simulink model "ControlSemCanalslx"  (Simulink 7.2)
settings: Solver=ode1  StartTime=0.0  StopTime=2  FixedStep=Ts  RelTol=1e-3
values from neighbouring files (symbols this model uses):
  C = [1 0]    [PIexp1.mat]    (also in PIexp3.mat; PIexp4.mat; PIpertubado.mat; ProjetoControlPI.m = GYzss.C)
  F = [621.187048977 29.8812144134]    [PIexp1.mat]    (also in PIexp3.mat; PIexp4.mat; PIpertubado.mat; ProjetoControlPI.m = FKi(1:size(G,2)))
  G = [1  0.0120914439825; 0  0.863556887172]    [PIexp1.mat]    (also in PIexp3.mat; PIexp4.mat; PIpertubado.mat; ProjetoControlPI.m = GYzss.A)
  H = [9.60922939797e-05 0.014430735648]    [PIexp1.mat]    (also in PIexp3.mat; PIexp4.mat; PIpertubado.mat; ProjetoControlPI.m = GYzss.B)
  K_AMP = 1    [PIexp1.mat]    (also in PIexp3.mat; PIexp4.mat; PIpertubado.mat; SemCanalExp1.mat)
  K_EC = 2.27485440932e-05    [PIexp1.mat]    (also in PIexp3.mat; PIexp4.mat; PIpertubado.mat; SemCanalExp1.mat)
  K_EP = 0.00153398078789    [PIexp1.mat]    (also in PIexp3.mat; PIexp4.mat; PIpertubado.mat; SemCanalExp1.mat)
  Kc = 1    [PIexp1.mat]    (also in PIexp3.mat; PIexp4.mat; PIpertubado.mat; ProjetoControlPI.m = 1/Y(end))
  L = [1.86355688717 61.6742300141]    [PIexp1.mat]    (also in PIexp3.mat; PIexp4.mat; PIpertubado.mat; ProjetoControlPI.m = L')
  Ts = 0.013    [PIexp1.mat]    (also in PIexp3.mat; PIexp4.mat; PIpertubado.mat; ProjetoControlPI.m)
  VMAX_AMP = 12    [PIexp1.mat]    (also in PIexp3.mat; PIexp4.mat; PIpertubado.mat; SemCanalExp1.mat)
  VMAX_DAC = 10    [PIexp1.mat]    (also in PIexp3.mat; PIexp4.mat; PIpertubado.mat; SemCanalExp1.mat)
  X_LIM_ENABLE = 1    [PIexp1.mat]    (also in PIexp3.mat; PIexp4.mat; PIpertubado.mat; SemCanalExp1.mat)
  X_MAX = 0.3    [PIexp1.mat]    (also in PIexp3.mat; PIexp4.mat; PIpertubado.mat; SemCanalExp1.mat)
  X_MIN = -0.3    [PIexp1.mat]    (also in PIexp3.mat; PIexp4.mat; PIpertubado.mat; SemCanalExp1.mat)
undefined symbols (not defined in the file or in its folder): HIL, qc_get_step_size
libraries: quarc_library x5, simulink x2, simulink_extras x1
settings Model: Creator=castr  LastModifiedBy=Aluno  SimulationMode=external  CovMetricSettings=dwe  CovHtmlReporting=off  covSaveCumulativeToWorkspaceVar=off  CovSaveSingleToWorkspaceVar=off  ExtModeTrigDuration=50000
settings SolverCC: PositivePriorityOrder=on
settings DataIOCC: LimitDataPoints=off  SaveFormat=StructureWithTime
settings OptimizationCC: ExpressionDepthLimit=128
settings DebuggingCC: UnderspecifiedInitializationDetection=Simplified  MergeDetectMultiDrivingBlocksExec=error  SolverPrmCheckMsg=none  FcnCallInpInsideContextMsg=Enable All  StateNameClashWarn=none  StrictBusMsg=ErrorLevel1
settings HardwareCC: ProdIntDivRoundTo=Zero  ProdEndianess=LittleEndian  ProdHWDeviceType=Specified
settings RTWCC: SystemTargetFile=quarc_windows.tlc  TemplateMakefile=quarc_default_tmf  Description=QUARC Win32 Target  ProcessScript=quarc_windows_make_rtw_hook
settings STFCustomTargetCC: TargetPreCompLibLocation=C:\DOCUME~1\ALLUSE~1\DADOSD~1\QUARC\lib\2008b\windows\release  SystemTargetFile=quarc_windows.tlc
settings GRTTargetCC: TargetPreCompLibLocation=C:\DOCUME~1\ALLUSE~1\DADOSD~1\QUARC\lib\2008b\windows\release  CompOptLevelCompliant=off  MatFileLogging=off  ExtMode=on  ExtModeMexFile=quarc_comm

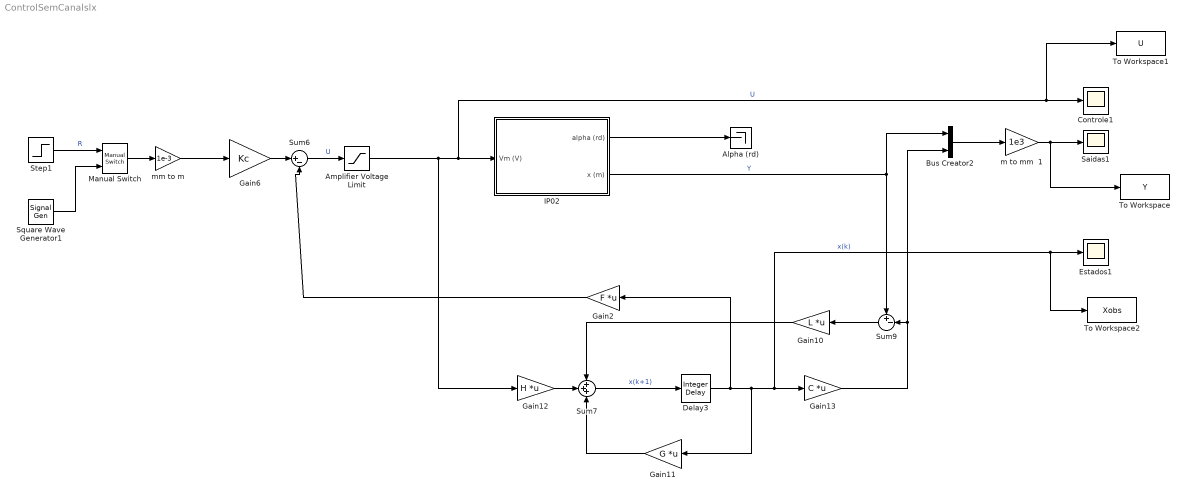
== system ControlSemCanalslx ==
  Alpha (rd) : Terminator
  Amplifier Voltage Limit : Saturate  UpperLimit=VMAX_AMP  LowerLimit=- VMAX_AMP  SampleTime=Ts
  Bus Creator2 : BusCreator  Inputs=2
  Controle1 : Scope
      settings: YMin=-1.5  YMax=13.5
  Delay3 : simulink/Discrete/Integer Delay  vinit=0.0  samptime=Ts  NumDelays=1
  Estados1 : Scope
      settings: YMin=-0.06898  YMax=0.62082  SaveName=ScopeData2
  Gain10 : Gain  Orientation=left  Gain=L  Multiplication=Matrix(K*u)
  Gain11 : Gain  Orientation=left  Gain=G  Multiplication=Matrix(K*u)
  Gain12 : Gain  Gain=H  Multiplication=Matrix(K*u)
  Gain13 : Gain  Gain=C  Multiplication=Matrix(K*u)
  Gain2 : Gain  Orientation=left  Gain=F  Multiplication=Matrix(K*u)
  Gain6 : Gain  Gain=Kc
  IP02 : Subsystem
  Manual Switch : simulink/Signal Routing/Manual Switch  SystemSampleTime=-1  sw=1  action=0  varsize=off
  Saidas1 : Scope
      settings: YMin=-37.5  YMax=337.5  SaveName=ScopeData3
  Square Wave Generator1 : SignalGenerator  WaveForm=square  Amplitude=150  Frequency=1.5  Units=rad/sec
  Step1 : Step  After=15  SampleTime=0
  Sum6 : Sum  Inputs=|+-
  Sum7 : Sum  Inputs=+++
  Sum9 : Sum  Orientation=left  Inputs=+-|
  To Workspace : ToWorkspace  VariableName=Y  SampleTime=-1  SaveFormat=Structure
  To Workspace1 : ToWorkspace  VariableName=U  SampleTime=-1  SaveFormat=Structure
  To Workspace2 : ToWorkspace  VariableName=Xobs  SampleTime=-1  SaveFormat=Structure
  m to mm  1 : Gain  Gain=1e3  SaturateOnIntegerOverflow=on  OutDataTypeStr=Inherit: Same as input  ParamDataTypeStr=Inherit: Same as input
  mm to m : Gain  Gain=1e-3
  wires:
  Gain11/1 -> Sum7/3
  Sum7/1 -> Delay3/1  "x(k+1)"
  Gain10/1 -> Sum7/1
  IP02/2(x (m)) -> Bus Creator2/1, Sum9/1  "Y"
  Amplifier Voltage Limit/1 -> IP02/1(Vm (V)), Controle1/1, To Workspace1/1, Gain12/1  "U"
  Delay3/1 -> Gain2/1, Gain13/1, Estados1/1, To Workspace2/1, Gain11/1  "x(k)"
  Gain12/1 -> Sum7/2
  Gain13/1 -> Sum9/2, Bus Creator2/2
  Sum9/1 -> Gain10/1
  Gain2/1 -> Sum6/2
  mm to m/1 -> Gain6/1
  Manual Switch/1 -> mm to m/1
  Square Wave Generator1/1 -> Manual Switch/2
  Step1/1 -> Manual Switch/1  "R"
  Gain6/1 -> Sum6/1
  Sum6/1 -> Amplifier Voltage Limit/1  "U"
  Bus Creator2/1 -> m to mm  1/1
  m to mm  1/1 -> Saidas1/1, To Workspace/1
  IP02/1(alpha (rd)) -> Alpha (rd)/1

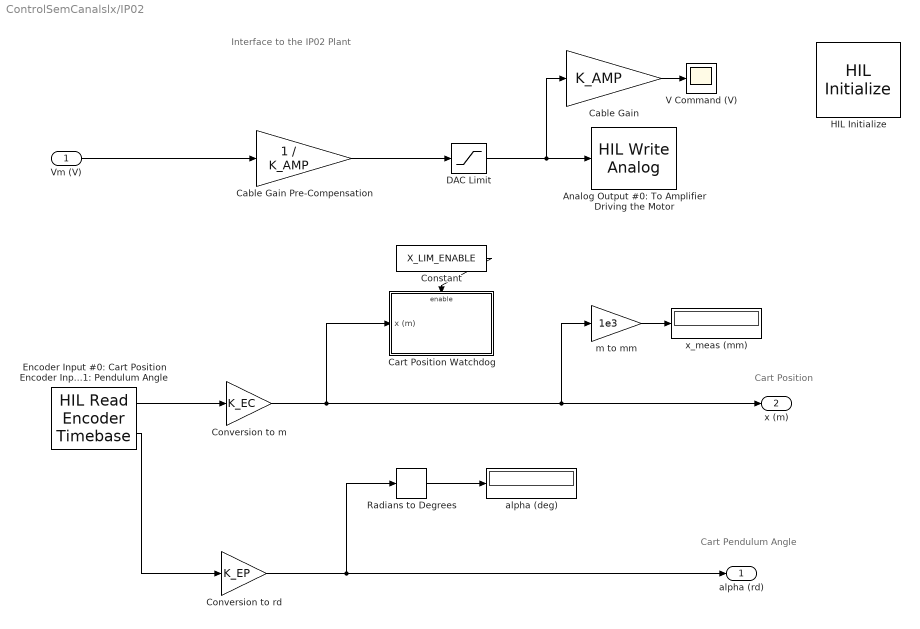
== system ControlSemCanalslx/IP02 ==
  note: Cart Pendulum Angle
  note: Cart Position
  note: Interface to the IP02 Plant
  Vm (V) : Inport
  Analog Output #0: To Amplifier Driving the Motor : quarc_library/Data Acquisition/Generic/Immediate I//O/HIL Write Analog  Tag=unassigned  object_name=HIL-1  channels=0  sample_time=-1  active=on  vector_input=on
  Cable Gain : Gain  Gain=K_AMP  SampleTime=Ts  SaturateOnIntegerOverflow=on  OutDataTypeStr=Inherit: Same as input  ParamDataTypeStr=Inherit: Same as input
  Cable Gain Pre-Compensation : Gain  Gain=1 / K_AMP  SampleTime=Ts  SaturateOnIntegerOverflow=on  OutDataTypeStr=Inherit: Same as input  ParamDataTypeStr=Inherit: Same as input
  Cart Position Watchdog : Subsystem  TreatAsAtomicUnit=on
  Constant : Constant  Value=X_LIM_ENABLE
  Conversion to m : Gain  Gain=K_EC  SampleTime=Ts  SaturateOnIntegerOverflow=on  OutDataTypeStr=Inherit: Same as input  ParamDataTypeStr=Inherit: Same as input
  Conversion to rd : Gain  Gain=K_EP  SampleTime=Ts  SaturateOnIntegerOverflow=on  OutDataTypeStr=Inherit: Same as input  ParamDataTypeStr=Inherit: Same as input
  DAC Limit : Saturate  UpperLimit=VMAX_DAC  LowerLimit=- VMAX_DAC  SampleTime=Ts
  Encoder Input #0: Cart Position Encoder Input #1: Pendulum Angle : quarc_library/Data Acquisition/Generic/Timebases/HIL Read Encoder Timebase  Tag=unassigned  object_name=HIL-1  clock=0  channels=[0,1]  samples_in_buffer=max(ceil(1/qc_get_step_size), 1)  active=on  vector_output=off  data_type_mode=Inherit via back propagation  data_type=double
  HIL Initialize : quarc_library/Data Acquisition/Generic/Configuration/HIL Initialize  object_name=HIL-1  board_type=q8_usb  board_number=0  board_options=update_rate=normal  exclusive=off  active=off  hardware_clocks=[0:2]  clock_modes=[]  set_clock_params_at_start=off  set_clock_params_at_switch_in=off  analog_input_channels=[0:7]  analog_input_maximums=10  analog_input_minimums=-10  set_analog_input_params_at_start=on  set_analog_input_params_at_switch_in=off  analog_output_channels=[0:7]  analog_output_maximums=10  analog_output_minimums=-10  initial_analog_outputs=[0]  final_analog_outputs=[0]  watchdog_analog_outputs=0  set_analog_output_params_at_start=on  set_analog_output_params_at_switch_in=off  set_analog_outputs_at_start=on  set_analog_outputs_at_switch_in=off  set_analog_outputs_at_terminate=on  set_analog_outputs_at_switch_out=off  set_analog_outputs_on_watchdog=off  digital_input_channels=[]  digital_output_channels=[0:7]  digital_output_configuration=[]  initial_digital_outputs=[0]  final_digital_outputs=[0]  watchdog_digital_outputs=[0]  set_digital_output_params_at_start=off  set_digital_output_params_at_switch_in=off  set_digital_outputs_at_start=on  set_digital_outputs_at_switch_in=off  set_digital_outputs_at_terminate=on  set_digital_outputs_at_switch_out=off  set_digital_outputs_on_watchdog=off  encoder_channels=[0:7]  quadrature=[4]  encoder_filter_frequency=[]  initial_encoder_counts=[0]  set_encoder_params_at_start=on  set_encoder_params_at_switch_in=off  set_encoder_counts_at_start=on  set_encoder_counts_at_switch_in=off  pwm_channels=[0:7]  pwm_modes=0  pwm_frequency=99.532799999999995e6/4095  pwm_configuration=[0]  pwm_alignment=[0]  pwm_polarity=[1]  pwm_leading_deadband=[0]  pwm_trailing_deadband=[0]  initial_pwm_outputs=[0]  final_pwm_outputs=[0]  watchdog_pwm_outputs=[0]  set_pwm_params_at_start=on  set_pwm_params_at_switch_in=off  set_pwm_outputs_at_start=on  set_pwm_outputs_at_switch_in=off  set_pwm_outputs_at_terminate=on  set_pwm_outputs_at_switch_out=off  set_pwm_outputs_on_watchdog=off  other_output_channels=[]  initial_other_outputs=[]  final_other_outputs=[]  watchdog_other_outputs=[]  set_other_outputs_at_start=off  set_other_outputs_at_switch_in=off  set_other_outputs_at_terminate=off  set_other_outputs_at_switch_out=off  set_other_outputs_on_watchdog=off
  Radians to Degrees : simulink_extras/Transformations/Radians to Degrees  SystemSampleTime=-1
  V Command (V) : Scope
      settings: TickLabels=on  TimeRange=5  YMin=-3  YMax=2.5  SaveName=data_vm  DataFormat=Array  MaxDataPoints=2500
  alpha (deg) : Display
      settings: Decimation=100
  m to mm : Gain  Gain=1e3  SampleTime=Ts  SaturateOnIntegerOverflow=on  OutDataTypeStr=Inherit: Same as input  ParamDataTypeStr=Inherit: Same as input
  x_meas (mm) : Display
      settings: Decimation=100
  alpha (rd) : Outport  InitialOutput=0
  x (m) : Outport  Port=2  InitialOutput=0
  wires:
  Encoder Input #0: Cart Position Encoder Input #1: Pendulum Angle/1 -> Conversion to m/1
  Conversion to m/1 -> Cart Position Watchdog/1(x (m)), x (m)/1, m to mm/1
  Cable Gain Pre-Compensation/1 -> DAC Limit/1
  m to mm/1 -> x_meas (mm)/1
  Encoder Input #0: Cart Position Encoder Input #1: Pendulum Angle/2 -> Conversion to rd/1
  Radians to Degrees/1 -> alpha (deg)/1
  Conversion to rd/1 -> Radians to Degrees/1, alpha (rd)/1
  Constant/1 -> Cart Position Watchdog/Enable
  DAC Limit/1 -> Analog Output #0: To Amplifier Driving the Motor/1, Cable Gain/1
  Vm (V)/1 -> Cable Gain Pre-Compensation/1
  Cable Gain/1 -> V Command (V)/1

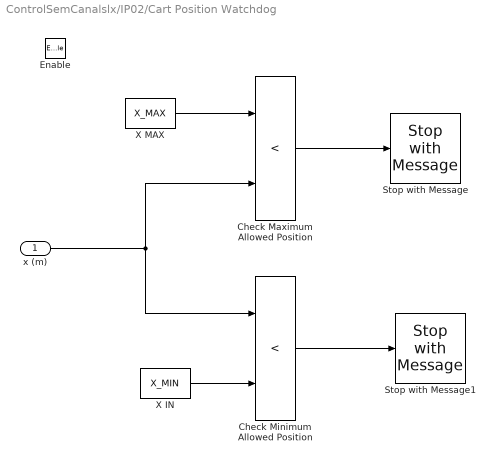
== system ControlSemCanalslx/IP02/Cart Position Watchdog ==
  x (m) : Inport
  Enable : EnablePort
  Check Maximum Allowed Position : RelationalOperator  Operator=<  InputSameDT=on
  Check Minimum Allowed Position : RelationalOperator  Operator=<  InputSameDT=on
  Stop with Message : quarc_library/Sinks/Error Handling/Stop with Message  SystemSampleTime=-1  message_type=Fixed error message  message_icon=Error  message=Maximum Limit Reached.
  Stop with Message1 : quarc_library/Sinks/Error Handling/Stop with Message  SystemSampleTime=-1  message_type=Fixed error message  message_icon=Error  message=Minimum Limit Reached.
  X IN : Constant  Value=X_MIN
  X MAX : Constant  Value=X_MAX
  wires:
  Check Maximum Allowed Position/1 -> Stop with Message/1
  x (m)/1 -> Check Minimum Allowed Position/1, Check Maximum Allowed Position/2
  X IN/1 -> Check Minimum Allowed Position/2
  Check Minimum Allowed Position/1 -> Stop with Message1/1
  X MAX/1 -> Check Maximum Allowed Position/1
